simulink model "projek2t"  (R2013a)
settings: Solver=ode45  SolverMode=SingleTasking  StartTime=0.0  StopTime=10.0  RelTol=1e-3
undefined symbols (not defined in the file): beta, In, J, Kp, Kt, Kw, lambdan, m, Mn, omegan, przelacz3, psien, R, regpred, T, Top, TR, Un, Uz0, V, Y
settings Model: Creator=user  LastModifiedBy=Jarek
settings DataIOCC: SignalLoggingSaveFormat=ModelDataLogs
settings OptimizationCC: BlockReduction=off  BooleanDataType=off
settings DebuggingCC: SaveWithParameterizedLinksMsg=none  SignalResolutionControl=TryResolveAllWithWarning  SolverPrmCheckMsg=none  MultiTaskDSMMsg=warning  MultiTaskCondExecSysMsg=none  StrictBusMsg=None
settings HardwareCC: TargetUnknown=on
settings RTWCC: IncludeERTFirstTime=on

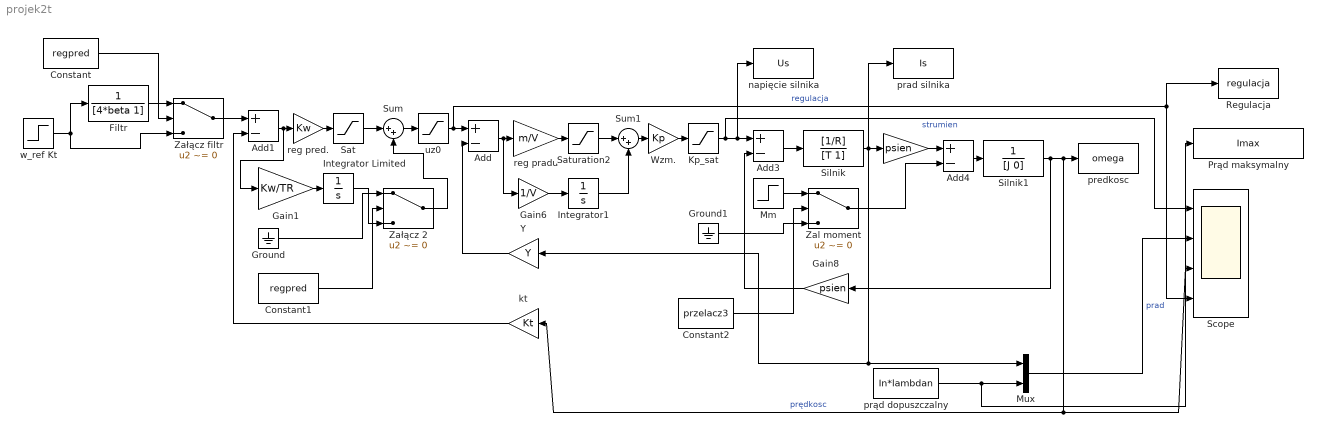
== system projek2t ==
  " " : Gain  Gain=psien
  Add{,1,3..4} (4 alike) : Sum  Inputs=+-
  Constant : Constant  Value=regpred
  Constant1 : Constant  Value=regpred
  Constant2 : Constant  Value=przelacz3
  Filtr : TransferFcn  Denominator=[4*beta 1]
  Gain1 : Gain  Gain=Kw/TR
  Gain6 : Gain  Gain=1/V
  Gain8 : Gain  Gain=psien
  Ground : Ground
  Ground1 : Ground
  Integrator Limited : Integrator  LimitOutput=on  UpperSaturationLimit=10  LowerSaturationLimit=-10
  Integrator1 : Integrator  LimitOutput=on  UpperSaturationLimit=10  LowerSaturationLimit=-10
  Kp_sat : Saturate  UpperLimit=1.5*Un  LowerLimit=-1.5*Un
  Mm : Step  Time=Top  After=Mn  SampleTime=0
  Mux : Mux  Inputs=2
  Prąd maksymalny : ToWorkspace  VariableName=Imax  SampleTime=-1  SaveFormat=Structure With Time
  Regulacja : ToWorkspace  VariableName=regulacja  SampleTime=-1  SaveFormat=Structure With Time
  Sat : Saturate  UpperLimit=10  LowerLimit=-10
  Saturation2 : Saturate  UpperLimit=10  LowerLimit=-10
  Scope : Scope  NumInputPorts=4
      settings: YMin=-5~-5~-5~-5  YMax=5~5~5~5
  Silnik : TransferFcn  Numerator=[1/R]  Denominator=[T 1]
  Silnik1 : TransferFcn  Denominator=[J 0]
  Sum : Sum  Inputs=|++
  Sum1 : Sum  Inputs=|++
  Wzm. : Gain  Gain=Kp
  Y : Gain  Gain=Y
  Zal moment : Switch  Criteria=u2 ~= 0
  Załącz 2 : Switch  Criteria=u2 ~= 0
  Załącz filtr : Switch  Criteria=u2 ~= 0
  kt : Gain  Gain=Kt
  napięcie silnika : ToWorkspace  VariableName=Us  SampleTime=-1  SaveFormat=Structure With Time
  prad silnika : ToWorkspace  VariableName=Is  SampleTime=-1  SaveFormat=Structure With Time
  predkosc : ToWorkspace  VariableName=omega  SampleTime=-1  SaveFormat=Structure With Time
  prąd dopuszczalny : Constant  Value=In*lambdan
  reg pradu : Gain  Gain=m/V
  "reg pred. " : Gain  Gain=Kw
  uz0 : Saturate  UpperLimit=Uz0  LowerLimit=-Uz0
  w_ref Kt : Step  Time=0  After=Kt*omegan  SampleTime=0
  wires:
  Add1/1 -> Gain1/1, "reg pred. "/1
  "reg pred. "/1 -> Sat/1
  Sat/1 -> Sum/1
  Gain1/1 -> Integrator Limited/1
  uz0/1 -> Scope/4, Regulacja/1, Add/1  "regulacja"
  reg pradu/1 -> Saturation2/1
  Add/1 -> Gain6/1, reg pradu/1
  Saturation2/1 -> Sum1/1
  Sum/1 -> uz0/1
  Sum1/1 -> Wzm./1
  Wzm./1 -> Kp_sat/1
  Kp_sat/1 -> Scope/1, napięcie silnika/1, Add3/1  "strumien"
  Gain6/1 -> Integrator1/1
  Integrator1/1 -> Sum1/2
  kt/1 -> Add1/2
  Y/1 -> Add/2
  Add3/1 -> Silnik/1
  Add4/1 -> Silnik1/1
  Silnik1/1 -> kt/1, Scope/3, predkosc/1, Gain8/1  "prędkosc"
  Gain8/1 -> Add3/2
  Silnik/1 -> Mux/1, Y/1, prad silnika/1, " "/1
  Mux/1 -> Scope/2  "prad"
  " "/1 -> Add4/1
  prąd dopuszczalny/1 -> Prąd maksymalny/1, Mux/2
  Załącz filtr/1 -> Add1/1
  w_ref Kt/1 -> Załącz filtr/3, Filtr/1
  Constant/1 -> Załącz filtr/2
  Załącz 2/1 -> Sum/2
  Constant1/1 -> Załącz 2/2
  Mm/1 -> Zal moment/1
  Zal moment/1 -> Add4/2
  Constant2/1 -> Zal moment/2
  Ground1/1 -> Zal moment/3
  Integrator Limited/1 -> Załącz 2/3
  Ground/1 -> Załącz 2/1
  Filtr/1 -> Załącz filtr/1
